simulink model "CombinedWithH2andBat"  (R2021a)
settings: Solver=VariableStepAuto  StartTime=0.0  StopTime=30*60*60  RelTol=1e-3
values from neighbouring files (symbols this model uses):
  A = length_of_wing^2*3.14 * number_of_windturbines    (= 78.5)    [load_global_variables.m]
  Area_panels = 700    [load_global_variables.m]
  Battery_Capacity = 10000    [load_global_variables.m]
  Efficiency_solar = 0.1    [load_global_variables.m]
  Efficiency_wind = 0.4    [load_global_variables.m]
  fuel_cell_power_rating = 5000    [load_global_variables.m]
  Max_H2_P_Input = 260000000    [load_global_variables.m]
  maxSOC = 95    [load_global_variables.m]
  Min_H2_P_Input = 1400    [load_global_variables.m]
  minSOC = 5    [load_global_variables.m]
  number_households = 200000    [load_global_variables.m]
  Rho = 1.204    [load_global_variables.m]
  SOC_Start = 50    [load_global_variables.m]
  Start_Tank_Fill_L = 1000000    [load_global_variables.m]
undefined symbols (not defined in the file or in its folder): Ion, Lithium, price, solarOneDay, time, wind
libraries: spsIdealSwitchLib x4, spsBatteryLib x1, spsDCVoltageSourceLib x1, spsSeriesRLCLoadLib x1, spspowerguiLib x1
settings Model: Creator=cm  LastModifiedBy=cm

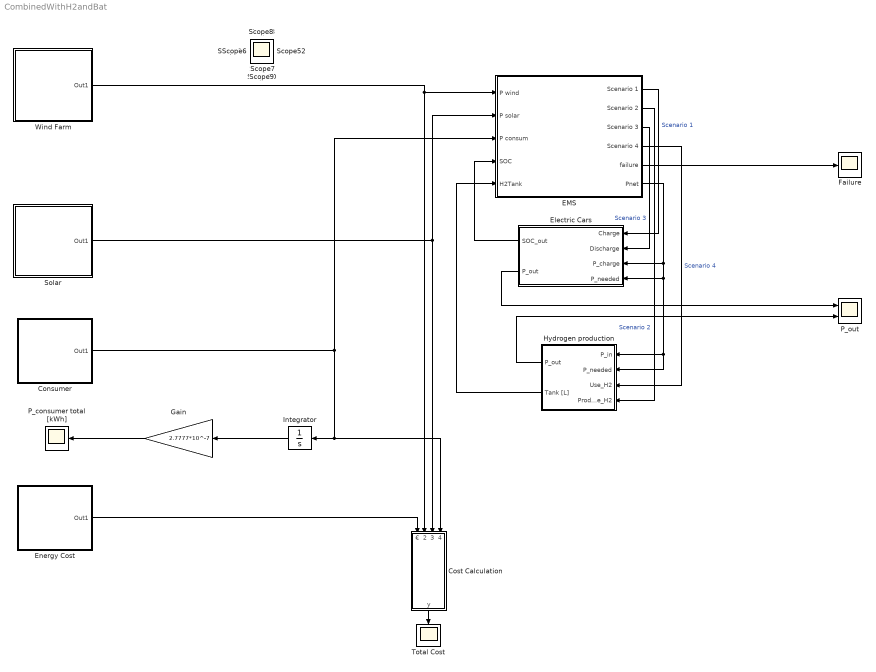
== system CombinedWithH2andBat ==
  Consumer : Subsystem
      mask Display: image('C:\Users\cm\OneDrive - Danmarks Tekniske Universitet\Model-Based Systems Eng\05 Models\MBSE-MicroGrid\OurModel\Icons\House.png'); % Use "Edit Image" on toolstrip to change.
  Cost Calculation : Subsystem
  EMS : Subsystem
  Electric Cars : Subsystem
  Energy Cost : Subsystem
      mask Display: image('C:\Users\cm\OneDrive - Danmarks Tekniske Universitet\Model-Based Systems Eng\05 Models\MBSE-MicroGrid\OurModel\Icons\el_cost.png'); % Use "Edit Image" on toolstrip to change.
  Failure : Scope
  Gain : Gain  Gain=2.7777*10^-7
  Hydrogen production : Subsystem
  Integrator : Integrator
  P_consumer total [kWh] : Scope
  P_out : Scope  NumInputPorts=2
  Solar : Subsystem
      mask Display: image('C:\Users\cm\OneDrive - Danmarks Tekniske Universitet\Model-Based Systems Eng\05 Models\MBSE-MicroGrid\OurModel\Icons\solar.png'); % Use "Edit Image" on toolstrip to change.
  Total Cost : Scope
  Wind Farm : Subsystem
      mask Display: image('C:\Users\cm\OneDrive - Danmarks Tekniske Universitet\Model-Based Systems Eng\05 Models\MBSE-MicroGrid\OurModel\Icons\wind.png'); % Use "Edit Image" on toolstrip to change.
  Scope{,1..10,12..13} (13 alike) : Scope
  wires:
  Wind Farm/1(Out1) -> EMS/1(P wind), Cost Calculation/2(P wind)
  Solar/1(Out1) -> Cost Calculation/3(P solar), EMS/2(P solar)
  Consumer/1(Out1) -> Cost Calculation/4(P_consumer), Integrator/1, EMS/3(P consum)
  Energy Cost/1(Out1) -> Cost Calculation/1(€)
  Cost Calculation/1(y) -> Total Cost/1
  EMS/1(Scenario 1) -> Electric Cars/1(Charge)  "Scenario 1"
  EMS/3(Scenario 3) -> Electric Cars/2(Discharge)  "Scenario 3"
  Integrator/1 -> Gain/1
  Gain/1 -> P_consumer total [kWh]/1
  Electric Cars/1(SOC_out) -> EMS/4(SOC)
  EMS/5(failure) -> Failure/1
  EMS/6(Pnet) -> Electric Cars/4(P_needed), Hydrogen production/1(P_in), Hydrogen production/2(P_needed), Electric Cars/3(P_charge)
  Hydrogen production/1(P_out) -> P_out/2
  Electric Cars/2(P_out) -> P_out/1
  Hydrogen production/2(Tank [L]) -> EMS/5(H2Tank)
  EMS/2(Scenario 2) -> Hydrogen production/4(Produce_H2)  "Scenario 2"
  EMS/4(Scenario 4) -> Hydrogen production/3(Use_H2)  "Scenario 4"

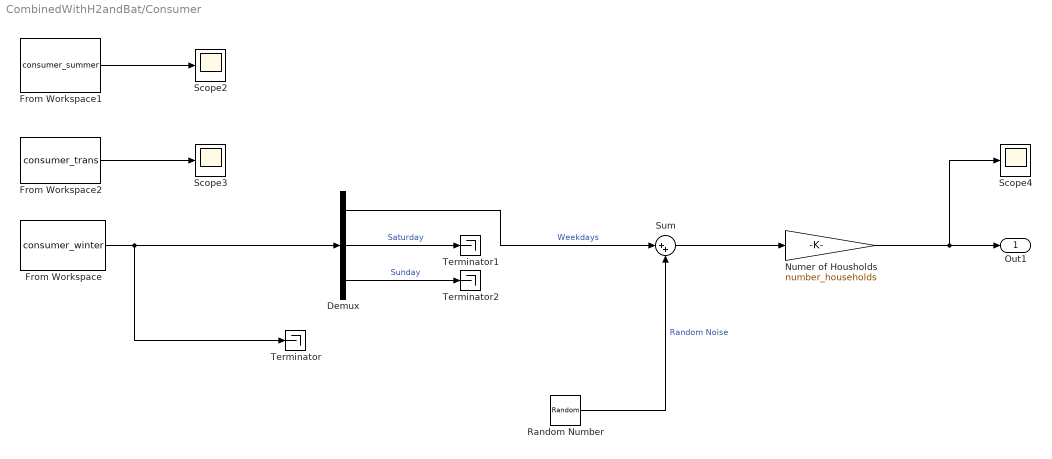
== system CombinedWithH2andBat/Consumer ==
  Demux : Demux  Outputs=3
  From Workspace : FromWorkspace  VariableName=consumer_winter  SampleTime=24*60*60/96  Interpolate=off  ZeroCross=off  OutputAfterFinalValue=Cyclic repetition
  From Workspace1 : FromWorkspace  VariableName=consumer_summer  SampleTime=24/96  Interpolate=off  ZeroCross=off  OutputAfterFinalValue=Cyclic repetition
  From Workspace2 : FromWorkspace  VariableName=consumer_trans  SampleTime=24/96  Interpolate=off  ZeroCross=off  OutputAfterFinalValue=Cyclic repetition
  Numer of Housholds : Gain  Gain=number_households
  Random Number : RandomNumber  Variance=0.0001  SampleTime=1*60*60
  Scope2 : Scope
  Scope3 : Scope
  Scope4 : Scope
  Sum : Sum  Inputs=|++
  Terminator : Terminator
  Terminator1 : Terminator
  Terminator2 : Terminator
  Out1 : Outport
  wires:
  Demux/2 -> Terminator1/1  "Saturday"
  From Workspace/1 -> Terminator/1, Demux/1
  From Workspace2/1 -> Scope3/1
  Random Number/1 -> Sum/2  "Random Noise"
  Demux/3 -> Terminator2/1  "Sunday"
  Sum/1 -> Numer of Housholds/1
  From Workspace1/1 -> Scope2/1
  Demux/1 -> Sum/1  "Weekdays"
  Numer of Housholds/1 -> Out1/1, Scope4/1

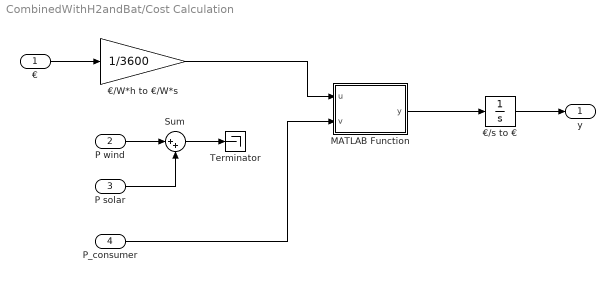
== system CombinedWithH2andBat/Cost Calculation ==
  € : Inport
  P wind : Inport  Port=2
  P solar : Inport  Port=3
  P_consumer : Inport  Port=4
  MATLAB Function : MATLAB Function  TreatAsAtomicUnit=on
  Sum : Sum  Inputs=|++
  Terminator : Terminator
  €/W*h to €/W*s : Gain  Gain=1/3600
  €/s to € : Integrator
  y : Outport
  wires:
  P wind/1 -> Sum/1
  P solar/1 -> Sum/2
  MATLAB Function/1(y) -> €/s to €/1
  €/W*h to €/W*s/1 -> MATLAB Function/1(u)
  €/1 -> €/W*h to €/W*s/1
  €/s to €/1 -> y/1
  Sum/1 -> Terminator/1
  P_consumer/1 -> MATLAB Function/2(v)

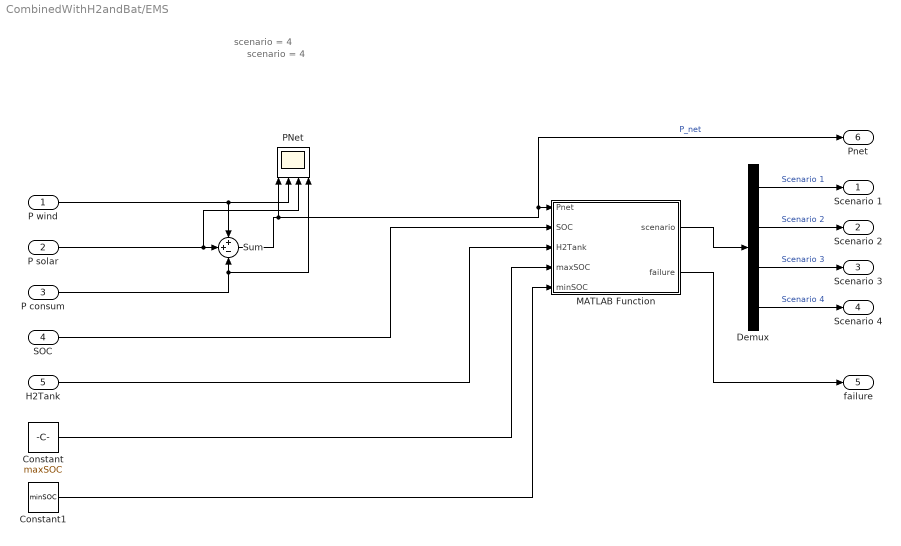
== system CombinedWithH2andBat/EMS ==
  note: scenario = 4
  note: scenario = 4
  P wind : Inport
  P solar : Inport  Port=2
  P consum : Inport  Port=3
  SOC : Inport  Port=4
  H2Tank : Inport  Port=5
  Constant : Constant  Value=maxSOC
  Constant1 : Constant  Value=minSOC
  Demux : Demux
  MATLAB Function : MATLAB Function  TreatAsAtomicUnit=on
  PNet : Scope  NumInputPorts=4
  Sum : Sum  Inputs=++-
  Scenario 1 : Outport
  Scenario 2 : Outport  Port=2
  Scenario 3 : Outport  Port=3
  Scenario 4 : Outport  Port=4
  failure : Outport  Port=5
  Pnet : Outport  Port=6
  wires:
  P wind/1 -> PNet/2, Sum/1
  Sum/1 -> Pnet/1, MATLAB Function/1(Pnet), PNet/1  "P_net"
  SOC/1 -> MATLAB Function/2(SOC)
  MATLAB Function/1(scenario) -> Demux/1
  Demux/1 -> Scenario 1/1  "Scenario 1"
  Demux/2 -> Scenario 2/1  "Scenario 2"
  Demux/3 -> Scenario 3/1  "Scenario 3"
  Demux/4 -> Scenario 4/1  "Scenario 4"
  P consum/1 -> PNet/4, Sum/3
  P solar/1 -> PNet/3, Sum/2
  H2Tank/1 -> MATLAB Function/3(H2Tank)
  MATLAB Function/2(failure) -> failure/1
  Constant/1 -> MATLAB Function/4(maxSOC)
  Constant1/1 -> MATLAB Function/5(minSOC)

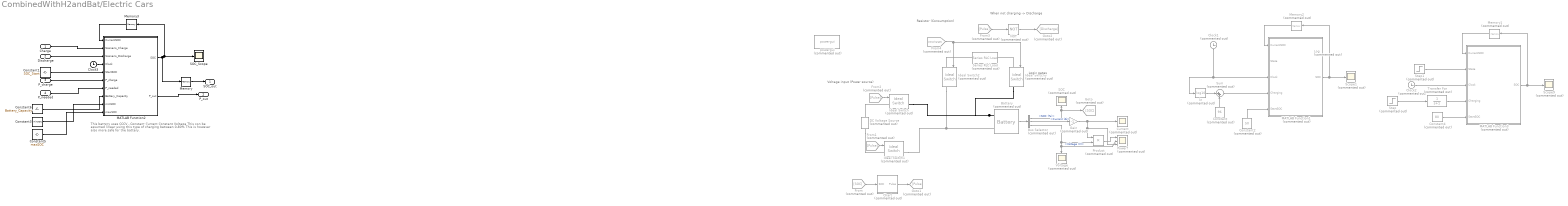
== system CombinedWithH2andBat/Electric Cars ==
  note: This battery uses CCCV - Constant Current Constant Voltage
      | This can be assumed linear using this type of charging between 0-80%
      | This is however also more safe for the battery.
  note: When not charging -> Discharge
  note: Logic gates
  note: Resistor (Consumption)
  note: Voltage input (Power source)
  Charge : Inport
  Discharge : Inport  Port=2
  P_charge : Inport  Port=3
  P_needed : Inport  Port=4
  Battery : spsBatteryLib/Battery  Commented=on  BatType=Lithium-Ion  ShowTempParam=off  ThermalPreset=no  ShowAgeParam=off  NomV=22.8  NomQ=230  SOC=0  Batt_Tr=30  PresetModel=on  MaxQ=230  MinV=17.1  FullV=26.5389  Dis_rate=100  R=0.0009913  Normal_OP=208  expZone="[24.6328         11.3]"  current=[6.5 13 32.5]  Units=Time  Tci=20  NomT=20  T2=-30  MaxQ2=4.8  FullV2=7.1  Normal_OP2=5.655  expZone2="[6.58           1]"  Rca=0.6  ti=2000  Dp=0  Neq0=0  Tsim=1e6  Ta1=25  Qeol=5.4*0.9  Reol=0.013333*1.2  Char_age=[2.3478, 3]  Dis_age=[2.3478, 10]  N1=1500  N2=10500  N3=1000  N4=1400  Ta2=45  N5=950
  Bus Selector : BusSelector  Commented=on  OutputSignals=SOC (%),Current (A),Voltage (V)
  Chart : Stateflow chart  Commented=on  TreatAsAtomicUnit=on
  Clock1 : Clock  Commented=on
      settings: Decimation=100
  Clock2 : Clock  Commented=on
      settings: Decimation=100
  Clock3 : Clock
      settings: Decimation=100
  Constant : Constant  Commented=on  Value=96
  Constant1 : Constant  Value=SOC_Start
  Constant2 : Constant  Commented=on  Value=50
  Constant3 : Constant  Value=minSOC
  Constant4 : Constant  Commented=on  Value=80
  Constant5 : Constant  Value=maxSOC
  Constant6 : Constant  Value=Battery_Capacity
  Current : Scope  Commented=on
  DC Voltage Source : spsDCVoltageSourceLib/DC Voltage Source  Commented=on  Amplitude=230  Measurements=None
  From : From  Commented=on  GotoTag=SOC
  From1 : From  Commented=on  GotoTag=Pulse
  From2 : From  Commented=on  GotoTag=Pulse
  From3 : From  Commented=on  GotoTag=Pulse
  From4 : From  Commented=on  GotoTag=Discharge
  Gain : Gain  Commented=on  Gain=-1
  Goto : Goto  Commented=on  GotoTag=SOC
  Goto1 : Goto  Commented=on  GotoTag=Pulse
  Goto2 : Goto  Commented=on  GotoTag=Discharge
  Ideal Switch{,1..3} (4 alike) : spsIdealSwitchLib/Ideal Switch  Commented=on  Ron=0.001  Lon=0  IC=0  Rs=1e5  Cs=inf  Measurements=on
  Log : Math  Commented=on  Operator=log  SaturateOnIntegerOverflow=on
  MATLAB Function1 : MATLAB Function  Commented=on  TreatAsAtomicUnit=on
  MATLAB Function2 : MATLAB Function  TreatAsAtomicUnit=on
  MATLAB Function3 : MATLAB Function  Commented=on  TreatAsAtomicUnit=on
  Memory : Memory  InheritSampleTime=on
  Memory1 : Memory  Commented=on  InheritSampleTime=on
  Memory2 : Memory  Commented=on  InheritSampleTime=on
  Memory3 : Memory  InheritSampleTime=on
  NOT : Logic  Commented=on  Operator=NOT  IconShape=distinctive  AllPortsSameDT=off  OutDataTypeStr=boolean
  Power? : Scope  Commented=on  NumInputPorts=3
  Product : Product  Commented=on
  SOC : Scope  Commented=on
  SOC_Scope : Scope
  Scope1 : Scope  Commented=on
  Scope9 : Scope  Commented=on
  Series RLC Load : spsSeriesRLCLoadLib/Series RLC Load  Commented=on  LConnTagsString=a  RConnTagsString=__new0  NominalVoltage=10  NominalFrequency=60  ActivePower=10e3  InductivePower=0  CapacitivePower=0  Setx0=off  InitialVoltage=0  SetiL0=off  InitialCurrent=0  Measurements=None  LoadType=constant Z
  Step : Step  Commented=on  Before=80  After=100  SampleTime=0
  Step1 : Step  Commented=on  Time=10  SampleTime=0
  Sum : Sum  Commented=on  Inputs=|++
  Transfer Fcn : TransferFcn  Commented=on  Denominator=[1 1]
  Voltage : Scope  Commented=on
  ln : Math  Commented=on  Operator=log10  SaturateOnIntegerOverflow=on
  powergui : spspowerguiLib/powergui  Priority=1  Commented=on  SimulationMode=Continuous  SampleTime=50e-6  frequency=60  Iterations=50  frequencyindice=0  Pbase=100e6  ErrMax=1e-4  UnitsV=kV  UnitsW=MW  buscounter=0  FunctionMessages=off  echomessages=off  EnableUseOfTLC=off  CurrentSourceSwitches=off  DisableSnubberDevices=off  DisableRonSwitches=off  DisableVfSwitches=off  DisplayEquations=off  AutomaticDiscreteSolvers=off  SolverType=Tustin/Backward Euler (TBE)  Interpol=off  ExternalGateDelay=off  methode=off  Ts=100  x0status=blocks  SPID=on  SwTol=0  HookPort=off  NonlinearTolerance=1e-4  nMaxIteration=100  ContinueOnMaxIteration=off  RestoreLinks=warning  ResistiveCurrentMeasurement=off  Frange=[0:2:500]  Ylog=off  Xlog=on  ShowGrid=off  save=off  variable=ZData  structure=0  ZoomFFT=off  StartTime=0.0  cycles=1  DisplayStyle=1  fundamental=60  FreqAxis=off  MaxFrequency=1000  frequencyindicesteady=1  RmsSteady=1  display=off
  SOC_out : Outport
  P_out : Outport  Port=2
  wires:
  Battery/1 -> Bus Selector/1
  From2/1 -> Ideal Switch/1
  Bus Selector/2 -> Gain/1  "<Current (A)>"
  From/1 -> Chart/1(SOC)
  From1/1 -> Ideal Switch1/1
  Bus Selector/3 -> Product/2, Power?/2, Voltage/1  "<Voltage (V)>"
  From4/1 -> Ideal Switch3/1, Ideal Switch2/1
  NOT/1 -> Goto2/1
  Bus Selector/1 -> Goto/1, SOC/1  "<SOC (%)>"
  Chart/1(Pulse) -> Goto1/1
  Product/1 -> Power?/1
  From3/1 -> NOT/1
  Gain/1 -> Power?/3, Product/1, Current/1
  Constant4/1 -> MATLAB Function3/5(StartSOC)
  MATLAB Function3/1(SOC) -> Scope9/1, Memory1/1
  Clock2/1 -> MATLAB Function3/3(Clock)
  Memory1/1 -> MATLAB Function3/1(CurrentSOC)
  Step/1 -> Transfer Fcn/1
  Transfer Fcn/1 -> MATLAB Function3/4(Charging)
  Step1/1 -> MATLAB Function3/2(State)
  ln/1 -> Sum/1
  MATLAB Function1/1(SOC) -> Memory2/1, Scope1/1
  Clock1/1 -> ln/1, MATLAB Function1/3(Clock)
  Memory2/1 -> MATLAB Function1/1(CurrentSOC)
  Constant2/1 -> MATLAB Function1/5(StartSOC)
  Sum/1 -> MATLAB Function1/4(Charging)
  Constant/1 -> Sum/2
  Clock3/1 -> MATLAB Function2/4(Clock)
  Constant1/1 -> MATLAB Function2/5(StartSOC)
  MATLAB Function2/1(SOC) -> SOC_Scope/1, Memory3/1, Memory/1
  Memory3/1 -> MATLAB Function2/1(CurrentSOC)
  Charge/1 -> MATLAB Function2/2(Scenario_Charge)
  Discharge/1 -> MATLAB Function2/3(Scenario_Discharge)
  MATLAB Function2/2(P_out) -> P_out/1
  Memory/1 -> SOC_out/1
  Constant3/1 -> MATLAB Function2/9(minSOC)
  Constant5/1 -> MATLAB Function2/10(maxSOC)
  Constant6/1 -> MATLAB Function2/8(Battery_Capacity)
  P_charge/1 -> MATLAB Function2/6(P_charge)
  P_needed/1 -> MATLAB Function2/7(P_needed)
  connections:
  Ideal Switch2/RConn1 -- Ideal Switch1/RConn1 -- Battery/LConn1
  Battery/LConn2 -- Ideal Switch/RConn1 -- Ideal Switch3/RConn1
  Ideal Switch3/LConn1 -- Series RLC Load/RConn1
  Ideal Switch2/LConn1 -- Series RLC Load/LConn1
  DC Voltage Source/LConn1 -- Ideal Switch/LConn1
  DC Voltage Source/RConn1 -- Ideal Switch1/LConn1

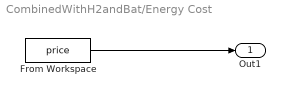
== system CombinedWithH2andBat/Energy Cost ==
  From Workspace : FromWorkspace  VariableName=price  SampleTime=24*60*60/length(price.signals.values)  Interpolate=off  ZeroCross=off  OutputAfterFinalValue=Cyclic repetition
  Out1 : Outport
  wires:
  From Workspace/1 -> Out1/1

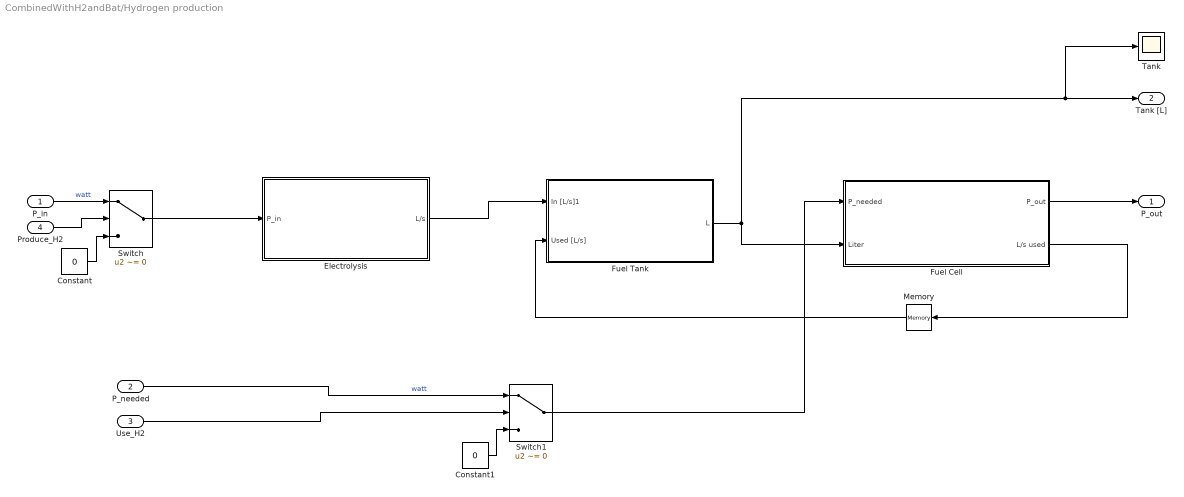
== system CombinedWithH2andBat/Hydrogen production ==
  P_in : Inport
  P_needed : Inport  Port=2
  Use_H2 : Inport  Port=3
  Produce_H2 : Inport  Port=4
  Constant : Constant  Value=0
  Constant1 : Constant  Value=0
  Electrolysis : Subsystem
  Fuel Cell : Subsystem
  Fuel Tank : Subsystem
  Memory : Memory
  Switch : Switch  Criteria=u2 ~= 0  Threshold=1
  Switch1 : Switch  Criteria=u2 ~= 0  Threshold=1
  Tank : Scope
  P_out : Outport
  Tank [L] : Outport  Port=2
  wires:
  Fuel Tank/1(L) -> Fuel Cell/2(Liter), Tank/1, Tank [L]/1
  Electrolysis/1(L/s) -> Fuel Tank/1(In [L/s]1)
  Fuel Cell/2(L/s used) -> Memory/1
  Fuel Cell/1(P_out) -> P_out/1
  Constant/1 -> Switch/3
  P_in/1 -> Switch/1  "watt"
  Switch/1 -> Electrolysis/1(P_in)
  Switch1/1 -> Fuel Cell/1(P_needed)
  Constant1/1 -> Switch1/3
  P_needed/1 -> Switch1/1  "watt"
  Produce_H2/1 -> Switch/2
  Use_H2/1 -> Switch1/2
  Memory/1 -> Fuel Tank/2(Used [L/s])

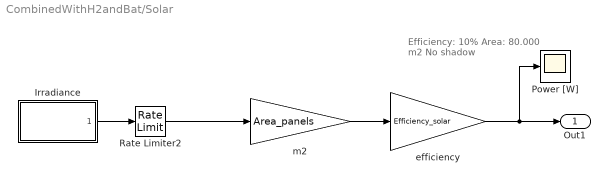
== system CombinedWithH2andBat/Solar ==
  note: Efficiency: 10%
      | Area: 80.000 m2
      | No shadow
  Irradiance : Subsystem
      mask init:
      | load power_V2G
      mask Display: plot(V2G.IRRADIANCE.time,V2G.IRRADIANCE.SUN)
  Power [W] : Scope
  Rate Limiter2 : RateLimiter  RisingSlewLimit=1e4  FallingSlewLimit=-1e4  SampleTimeMode=inherited
  efficiency : Gain  Gain=Efficiency_solar
  m2 : Gain  Gain=Area_panels
  Out1 : Outport
  wires:
  Irradiance/1(" ") -> Rate Limiter2/1
  m2/1 -> efficiency/1
  efficiency/1 -> Out1/1, Power [W]/1
  Rate Limiter2/1 -> m2/1

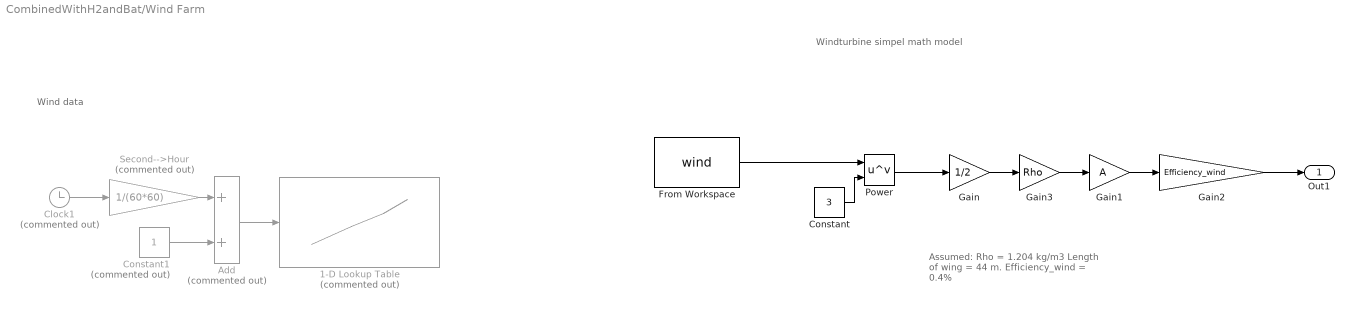
== system CombinedWithH2andBat/Wind Farm ==
  note: Assumed:
      | Rho = 1.204 kg/m3
      | Length of wing = 44 m.
      | Efficiency_wind = 0.4%
  note: Windturbine simpel math model
  note: Wind data
  1-D Lookup Table : Lookup_n-D  Commented=on  NumberOfTableDimensions=1  BreakpointsForDimension1=time  BeginIndexSearchUsingPreviousIndexResult=on  Table=wind  ExtrapMethod=Clip  UseLastTableValue=on  InternalRulePriority=Speed  RndMeth=Simplest  InputSameDT=on
  Add : Sum  Commented=on
  Clock1 : Clock  Commented=on
  Constant : Constant  Value=3
  Constant1 : Constant  Commented=on
  From Workspace : FromWorkspace  VariableName=wind  SampleTime=24*60*60/(length(wind.signals.values))  Interpolate=off  ZeroCross=off  OutputAfterFinalValue=Cyclic repetition
  Gain : Gain  Gain=1/2
  Gain1 : Gain  Gain=A
  Gain2 : Gain  Gain=Efficiency_wind
  Gain3 : Gain  Gain=Rho
  Power : Math  Operator=pow  SaturateOnIntegerOverflow=on
  Second-->Hour : Gain  Commented=on  Gain=1/(60*60)
  Out1 : Outport
  wires:
  Power/1 -> Gain/1
  Clock1/1 -> Second-->Hour/1
  Gain1/1 -> Gain2/1
  Second-->Hour/1 -> Add/1
  Add/1 -> 1-D Lookup Table/1
  Constant/1 -> Power/2
  Constant1/1 -> Add/2
  Gain/1 -> Gain3/1
  Gain3/1 -> Gain1/1
  Gain2/1 -> Out1/1
  From Workspace/1 -> Power/1

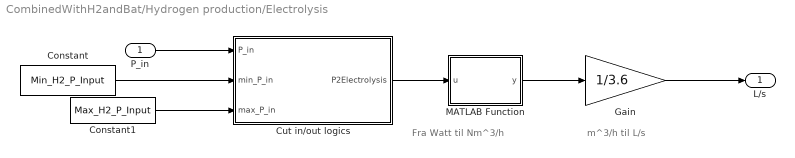
== system CombinedWithH2andBat/Hydrogen production/Electrolysis ==
  note: m^3/h til L/s
  note: Fra Watt til Nm^3/h
  P_in : Inport
  Constant : Constant  Value=Min_H2_P_Input
  Constant1 : Constant  Value=Max_H2_P_Input
  Cut in/out logics : MATLAB Function  TreatAsAtomicUnit=on
  Gain : Gain  Gain=1/3.6
  MATLAB Function : MATLAB Function  TreatAsAtomicUnit=on
  L/s : Outport
  wires:
  P_in/1 -> Cut in/out logics/1(P_in)
  Constant/1 -> Cut in/out logics/2(min_P_in)
  Constant1/1 -> Cut in/out logics/3(max_P_in)
  Cut in/out logics/1(P2Electrolysis) -> MATLAB Function/1(u)
  MATLAB Function/1(y) -> Gain/1
  Gain/1 -> L/s/1

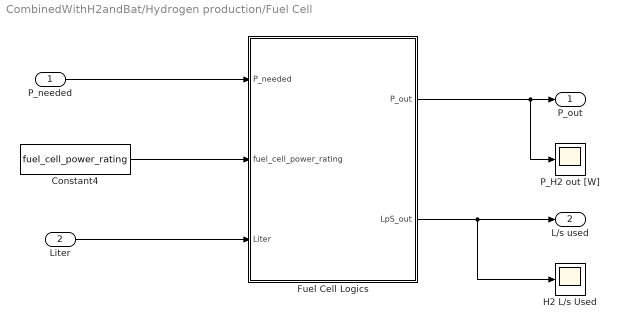
== system CombinedWithH2andBat/Hydrogen production/Fuel Cell ==
  P_needed : Inport
  Liter : Inport  Port=2
  Constant4 : Constant  Value=fuel_cell_power_rating
  Fuel Cell Logics : MATLAB Function  TreatAsAtomicUnit=on
  H2 L/s Used : Scope
  P_H2 out [W] : Scope
  P_out : Outport
  L/s used : Outport  Port=2
  wires:
  Constant4/1 -> Fuel Cell Logics/2(fuel_cell_power_rating)
  Fuel Cell Logics/1(P_out) -> P_H2 out [W]/1, P_out/1
  P_needed/1 -> Fuel Cell Logics/1(P_needed)
  Fuel Cell Logics/2(LpS_out) -> H2 L/s Used/1, L/s used/1
  Liter/1 -> Fuel Cell Logics/3(Liter)

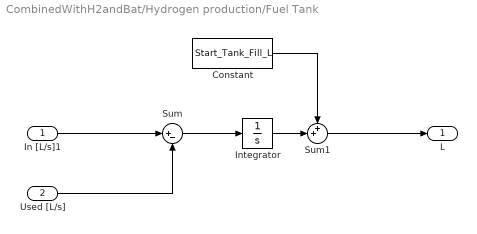
== system CombinedWithH2andBat/Hydrogen production/Fuel Tank ==
  In [L/s]1 : Inport
  Used [L/s] : Inport  Port=2
  Constant : Constant  Value=Start_Tank_Fill_L
  Integrator : Integrator
  Sum : Sum  Inputs=|+-
  Sum1 : Sum  Inputs=++|
  L : Outport
  wires:
  Used [L/s]/1 -> Sum/2
  In [L/s]1/1 -> Sum/1
  Sum/1 -> Integrator/1
  Constant/1 -> Sum1/1
  Integrator/1 -> Sum1/2
  Sum1/1 -> L/1

== system CombinedWithH2andBat/Solar/Irradiance ==
  From Workspace : FromWorkspace  VariableName=solar  SampleTime=24*60*60/(length(solarOneDay))  Interpolate=off  ZeroCross=off  OutputAfterFinalValue=Cyclic repetition
  " " : Outport  VectorParamsAs1DForOutWhenUnconnected=off
  wires:
  From Workspace/1 -> " "/1

== matlab function CombinedWithH2andBat/Hydrogen production/Fuel Cell/Fuel Cell Logics ==
  data: P_out output; P_needed input; fuel_cell_power_rating input; LpS_out output; Liter input
function [P_out,LpS_out]  = fcn(P_needed, fuel_cell_power_rating, Liter)


P_needed = abs(P_needed);
%Her omdaner vi fra H2 L til W
x1=0;
x2=0.22533333333;

y1=0;
y2=1;

a=(y2-y1)/(x2-x1);
b=y2-a*x1;

max_P_out_L =  (fuel_cell_power_rating-b)/ a;


if Liter > max_P_out_L
    if P_needed <= fuel_cell_power_rating
       P_out = P_needed;
    elseif P_needed > fuel_cell_power_rating
        P_out = fuel_cell_power_rating;
    else
        % not needed but to safe our butts
        error('In Fuel Cell: We got to a case which should not happen')
        P_out = P_needed;
    end

else 
    P_out = 0;
    
end



LpS_out = (P_needed-b)/ a;
    
end

== matlab function CombinedWithH2andBat/Cost Calculation/MATLAB Function ==
  data: u input; y output; v input
function y = multiply(u,v)

y = u*v;

== matlab function CombinedWithH2andBat/EMS/MATLAB Function ==
  data: Pnet input; scenario output; SOC input; H2Tank input; failure output; maxSOC input; minSOC input
function [scenario,failure] = fcn(Pnet,SOC,H2Tank,maxSOC,minSOC)
scenario = [0,0,0,0];
failure = 0;
if Pnet>0
    % more engery produced than consumed
   if SOC >= maxSOC 
       % Battery full
       if H2Tank >= 1000000000 %TODO: global var
           % H2 tank full
           failure = 1;
           disp('Overproduction');
       else
           % Poduce Hydrogen
            scenario = [0 1 0 0];
       end
   else
       % Battery not full
       scenario = [1 0 0 0]; % charge battery       
   end
else
    % more energy consumed than produced
    if SOC <= minSOC 
        % Battery empty
        if H2Tank <=0
            failure = 1;
            disp('Blackout')
        else
            % Use Hydrogen
            scenario = [0 0 0 1]; % TODO: define actions for case. No energy in system left
        end
    else
        % Battery not empty
        scenario = [0 0 1 0]; % discharge battery
    end
end

== stateflow chart CombinedWithH2andBat/Electric Cars/Chart ==
  state Charge
    entry : Pulse = 1
  state Discharge
    entry : Pulse = 0
  (default) -> Charge
  Charge -> Discharge : [SOC>80]
  Discharge -> Charge : [SOC<20]
  data: SOC input; Pulse output

== matlab function CombinedWithH2andBat/Electric Cars/MATLAB Function1 ==
  data: CurrentSOC input; SOC output; State input; Clock input; Charging input; StartSOC input
function SOC = fcn(CurrentSOC,State,Clock, Charging, StartSOC)




% if Clock > 30
%     
%     State = 1;
% 
% end 

% if Clock > 50
%     
%     State =2;
%     
% end

% if CurrentSOC < 50
%     
%     State = 1;
%     
% end

if State == 0 %Discharging
    if CurrentSOC <= 0
        SOC = 0;
    else
    SOC = CurrentSOC - 0.001;
    end
    
elseif State == 1 %Charging
    
    if CurrentSOC >= 100
        SOC = 100;
    elseif CurrentSOC < 95
        SOC = CurrentSOC + 0.01 %/ CurrentSOC;
    else
     SOC = Charging;
    end
else % Idle
    
    SOC =CurrentSOC;
    
end

if Clock == 0
    SOC = StartSOC;
end
    
end

== matlab function CombinedWithH2andBat/Electric Cars/MATLAB Function3 ==
  data: CurrentSOC input; SOC output; State input; Clock input; Charging input; StartSOC input
function SOC = fcn(CurrentSOC,State,Clock, Charging, StartSOC)




% if Clock > 30
%     
%     State = 1;
% 
% end 

% if Clock > 50
%     
%     State =2;
%     
% end

% if CurrentSOC < 50
%     
%     State = 1;
%     
% end

if State == 0 %Discharging
    if CurrentSOC == 0
        SOC = 0
    else
    
    SOC = CurrentSOC - 2;
    end
elseif State == 1 %Charging

 
     SOC = Charging;

else % Idle
    
    SOC =CurrentSOC;
    
end

if Clock == 0
    SOC = StartSOC;
end
    
end

== matlab function CombinedWithH2andBat/Electric Cars/MATLAB Function2 ==
  data: CurrentSOC input; SOC output; Scenario_Charge input; Scenario_Discharge input; Clock input; StartSOC input; P_charge input; P_out output; P_needed input; Battery_Capacity input; minSOC input; maxSOC input
function [SOC,P_out]= SOC(CurrentSOC,Scenario_Charge, Scenario_Discharge,Clock, StartSOC,...
                        P_charge, P_needed, Battery_Capacity, minSOC, maxSOC)


P_out = 0;


if Scenario_Discharge == 1 %Discharging
    if CurrentSOC <= minSOC
        SOC = minSOC;
    else
    SOC = CurrentSOC +P_needed/Battery_Capacity; % P_needed is negative
    P_out = P_needed;
    end
    
elseif Scenario_Charge == 1 %Charging
    
    if CurrentSOC >= maxSOC
        SOC = maxSOC;
    
    else 
        
        SOC = CurrentSOC + P_charge/Battery_Capacity;
        
    end



else % Idle
    
    SOC =CurrentSOC;
    
end

if Clock == 0
    SOC = StartSOC;
end
    
end

== matlab function CombinedWithH2andBat/Hydrogen production/Electrolysis/Cut in//out logics ==
  data: P_in input; min_P_in input; P2Electrolysis output; max_P_in input
function P2Electrolysis = fcn(P_in, min_P_in, max_P_in)

if P_in >= min_P_in && P_in <= max_P_in
    
    P2Electrolysis = P_in;
elseif P_in > max_P_in
    P2Electrolysis = max_P_in;
elseif P_in < min_P_in
    P2Electrolysis = 0;
else
    % case shouldnt happen, but to secure our butts
    P2Electrolysis = max_P_in;
end

== matlab function CombinedWithH2andBat/Hydrogen production/Electrolysis/MATLAB Function ==
  data: u input; y output
function y = fcn(u)
 
%Værdier for min og maks Elektrolyse 
% https://cellar-c2.services.clever-cloud.com/com-mcphy/uploads/2020/08/20.05.McPhy_Portfolio_ELY_Piel_EN.pdf
x2=26000000
x1=14000

y2=4.4*10
y1=2.4


a=(log(y2)-log(y1))/(log(x2)-log(x1))

b=y1/(x1^a)

y=b*u^a
